simulink model "LA_KF"  (R2022a)
settings: Solver=FixedStepAuto  StartTime=0.0  StopTime=10.0  RelTol=1e-3
values from neighbouring files (symbols this model uses):
  Arm_resistance = 2.2    [Ram_rollerm.m]
  C_scr = 1.2e3    (= 1200)    [Ram_rollerm.m]
  D = 8e-5    (= 8e-05)    [Ram_rollerm.m]
  h = l/(2*pi)    (= 0.000381971863421)    [Ram_rollerm.m]
  he = 0.05    [Ram_rollerm.m]
  J = 5.3e-5    (= 5.3e-05)    [Ram_rollerm.m]
  k = 500e6    (= 500000000)    [Ram_rollerm.m]
  Ke = 0.121    [Ram_rollerm.m]
  Km = 1e7    (= 10000000)    [Ram_rollerm.m]
  Ks = 1.8e5    (= 180000)    [Ram_rollerm.m]
  Kt = 0.121    [Ram_rollerm.m]
  La = 6.4e-3    (= 0.0064)    [Ram_rollerm.m]
  lqr_Lr = lqr(Plant.A,Plant.B,lqr_Q,lqr_R)    [Ram_rollerm.m]
  M_load = 20    [Ram_rollerm.m]
  M_scr = 2    [Ram_rollerm.m]
  mu = 0.3    [Ram_rollerm.m]
  n = 0.25    [Ram_rollerm.m]
  omega = 2*pi*rpm    (= 6.28318530718)    [Ram_rollerm.m]
  R = 0.1778    [Ram_rollerm.m]
  sysKF = ss(Plant.A-Kf*Plant.C,[Plant.B Kf],eye(7),0*[Plant.B Kf])    [Ram_rollerm.m]
  w = (wo + wf)/2    (= 0.1535)    [Ram_rollerm.m]
undefined symbols (not defined in the file or in its folder): Plant
settings Model: Creator=linda  LastModifiedBy=royka
settings DebuggingCC: UnconnectedInputMsg=warning  UnconnectedOutputMsg=warning  UnconnectedLineMsg=warning
settings RTWCC: DLArmComputeVersion=19.05

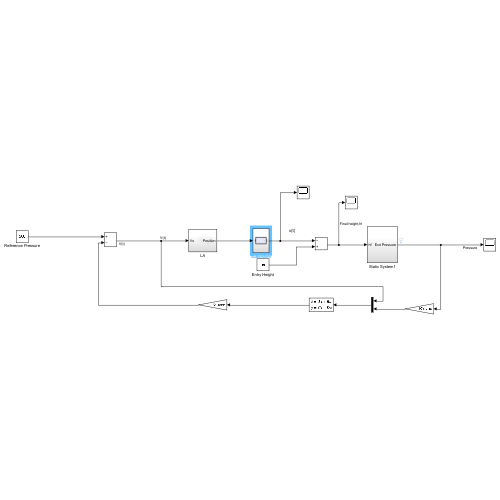
[thumbnail: Simulink's stored preview of the top-level diagram]
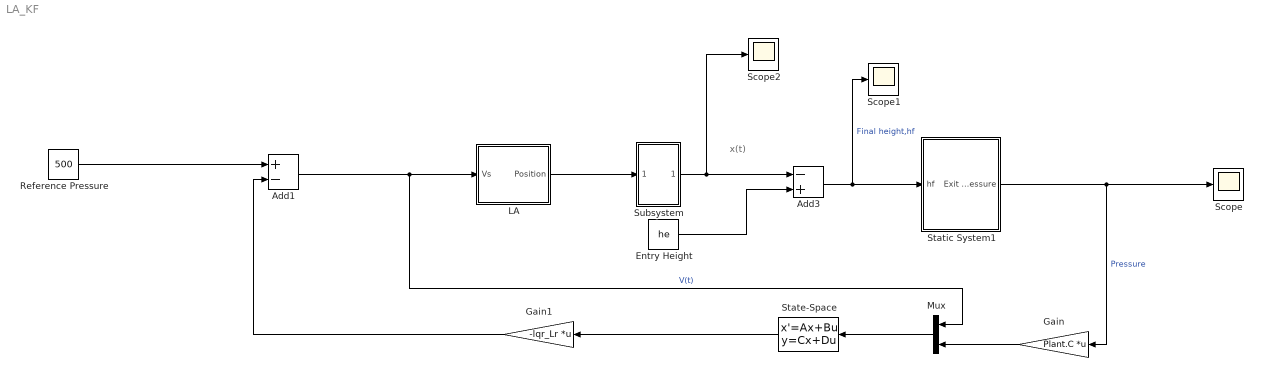
== system LA_KF ==
  note: x(t)
  Add1 : Sum  Inputs=+-
  Add3 : Sum  Inputs=-+
  Entry Height : Constant  Value=he
  Gain : Gain  Gain=Plant.C  Multiplication=Matrix(K*u) (u vector)
  Gain1 : Gain  Gain=-lqr_Lr  Multiplication=Matrix(K*u) (u vector)
  LA : Subsystem
  Mux : Mux  Inputs=2
  Reference Pressure : Constant  Value=500
  Scope : Scope
  Scope1 : Scope
  Scope2 : Scope
  State-Space : StateSpace  A=sysKF.A  B=sysKF.B  C=sysKF.C  D=sysKF.D  InitialCondition=0
  Static System1 : Subsystem
  Subsystem : Subsystem
  wires:
  Entry Height/1 -> Add3/2
  Static System1/1(Exit Pressure) -> Gain/1, Scope/1  "Pressure"
  Reference Pressure/1 -> Add1/1
  Add3/1 -> Scope1/1, Static System1/1(hf)  "Final height,hf"
  LA/1(Position) -> Subsystem/1(In1)
  Mux/1 -> State-Space/1
  Gain/1 -> Mux/2
  State-Space/1 -> Gain1/1
  Add1/1 -> LA/1(Vs), Mux/1  "V(t)"
  Gain1/1 -> Add1/2
  Subsystem/1(Out1) -> Scope2/1, Add3/1

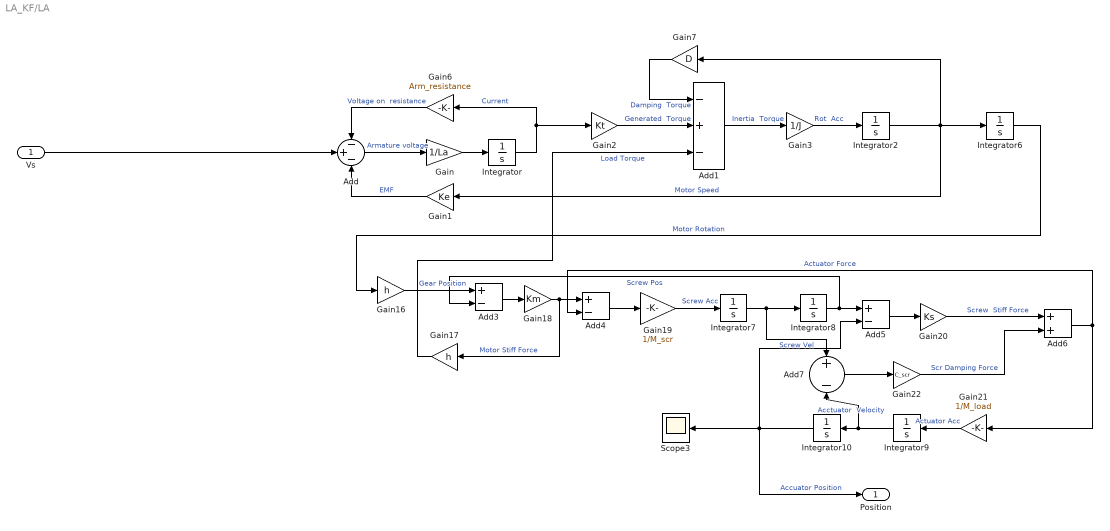
== system LA_KF/LA ==
  Vs : Inport
  Add : Sum  Inputs=-+-
  Add1 : Sum  Inputs=-+-
  Add{3..5,7} (4 alike) : Sum  Inputs=+-
  Add6 : Sum
  Gain : Gain  Gain=1/La
  Gain1 : Gain  Gain=Ke
  Gain16 : Gain  Gain=h
  Gain17 : Gain  Gain=h
  Gain18 : Gain  Gain=Km
  Gain19 : Gain  Gain=1/M_scr
  Gain2 : Gain  Gain=Kt
  Gain20 : Gain  Gain=Ks
  Gain21 : Gain  Gain=1/M_load
  Gain22 : Gain  Gain=C_scr
  Gain3 : Gain  Gain=1/J
  Gain6 : Gain  Gain=Arm_resistance
  Gain7 : Gain  Gain=D
  Integrator{,2,6..10} (7 alike) : Integrator
  Scope3 : Scope
  Position : Outport
  wires:
  Gain16/1 -> Add3/1  "Gear Position"
  Gain/1 -> Integrator/1
  Integrator8/1 -> Add3/2, Add5/1  "Screw Pos"
  Gain19/1 -> Integrator7/1  "Screw Acc"
  Gain2/1 -> Add1/2  "Generated  Torque"
  Gain20/1 -> Add6/1  "Screw  Stiff Force"
  Add1/1 -> Gain3/1  "Inertia  Torque"
  Vs/1 -> Add/2
  Gain17/1 -> Add1/3  "Load Torque"
  Gain1/1 -> Add/3  "EMF"
  Gain21/1 -> Integrator9/1  "Actuator Acc"
  Add/1 -> Gain/1  "Armature voltage"
  Add3/1 -> Gain18/1
  Gain22/1 -> Add6/2  "Scr Damping Force"
  Integrator9/1 -> Add7/2, Integrator10/1  "Acctuator  Velocity"
  Add7/1 -> Gain22/1
  Add5/1 -> Gain20/1
  Integrator/1 -> Gain6/1, Gain2/1  "Current"
  Gain6/1 -> Add/1  "Voltage on  resistance"
  Gain3/1 -> Integrator2/1  "Rot  Acc"
  Add6/1 -> Gain21/1, Add4/2  "Actuator Force"
  Integrator10/1 -> Position/1, Add5/2, Scope3/1  "Accuator Position"
  Add4/1 -> Gain19/1
  Integrator2/1 -> Gain1/1, Integrator6/1, Gain7/1  "Motor Speed"
  Integrator6/1 -> Gain16/1  "Motor Rotation"
  Gain7/1 -> Add1/1  "Damping  Torque"
  Integrator7/1 -> Add7/1, Integrator8/1  "Screw Vel"
  Gain18/1 -> Gain17/1, Add4/1  "Motor Stiff Force"

== system LA_KF/Static System1 ==
  hf : Inport
  Constant10 : Constant  Value=omega
  Subsystem : Subsystem
  Exit Pressure : Outport
  wires:
  hf/1 -> Subsystem/2(hf)  "hf"
  Constant10/1 -> Subsystem/1(omega)
  Subsystem/1(Out1) -> Exit Pressure/1

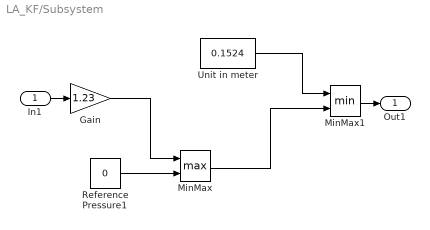
== system LA_KF/Subsystem ==
  In1 : Inport
  "Gain " : Gain  Gain=1.23
  MinMax : MinMax  Function=max  Inputs=2
  MinMax1 : MinMax  Inputs=2
  Reference Pressure1 : Constant  Value=0
  Unit in meter : Constant  Value=0.1524
  Out1 : Outport
  wires:
  MinMax1/1 -> Out1/1
  "Gain "/1 -> MinMax/1
  MinMax/1 -> MinMax1/2
  Unit in meter/1 -> MinMax1/1
  Reference Pressure1/1 -> MinMax/2
  In1/1 -> "Gain "/1

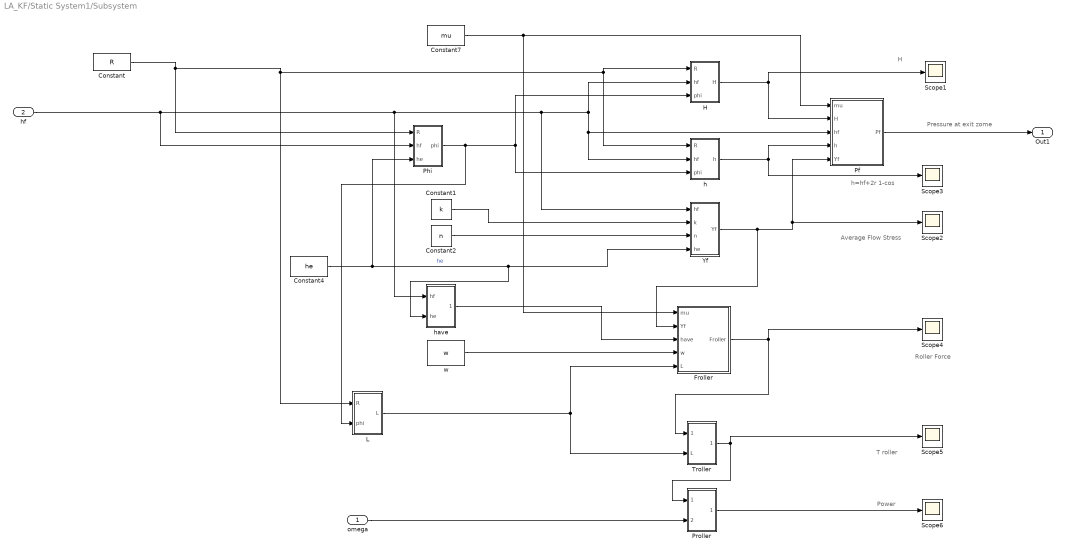
== system LA_KF/Static System1/Subsystem ==
  note: Power
  note: T roller
  note: Roller Force
  note: Pressure at exit zome
  note: h=hf+2r 1-cos
  note: Average Flow Stress
  note: H
  omega : Inport
  hf : Inport  Port=2
  Constant : Constant  Value=R
  Constant1 : Constant  Value=k
  Constant2 : Constant  Value=n
  Constant4 : Constant  Value=he
  Constant7 : Constant  Value=mu
  Froller : Subsystem
  H : Subsystem
  L : Subsystem
  Pf : Subsystem
  Phi : Subsystem
  Proller : Subsystem
  Scope{1..6} (6 alike) : Scope
  Troller : Subsystem
  Yf : Subsystem
  h : Subsystem
  have : Subsystem
  w : Constant  Value=w
  Out1 : Outport
  wires:
  omega/1 -> Proller/2(In2)
  hf/1 -> Phi/2(hf), Yf/1(hf), h/2(hf), Pf/3(hf), H/2(hf), have/1(hf)
  Yf/1(Yf) -> Froller/2(Yf), Scope2/1, Pf/5(Yf)
  Constant7/1 -> Froller/1(mu), Pf/1(mu)
  Proller/1(Out1) -> Scope6/1
  Constant4/1 -> Phi/3(he), have/2(he), Yf/4(he)  "he"
  h/1(h) -> Scope3/1, Pf/4(h)
  H/1(H) -> Scope1/1, Pf/2(H)
  w/1 -> Froller/4(w)
  Troller/1(Troller) -> Proller/1(In1), Scope5/1
  Constant2/1 -> Yf/3(n)
  Constant1/1 -> Yf/2(k)
  Froller/1(Froller) -> Scope4/1, Troller/1(Froller)
  Constant/1 -> Phi/1(R), L/1(R), H/1(R), h/1(R)
  Pf/1(Pf) -> Out1/1
  have/1(Out1) -> Froller/3(have)
  Phi/1(phi) -> L/2(phi), h/3(phi), H/3(phi)
  L/1(L) -> Troller/2(L), Froller/5(L)

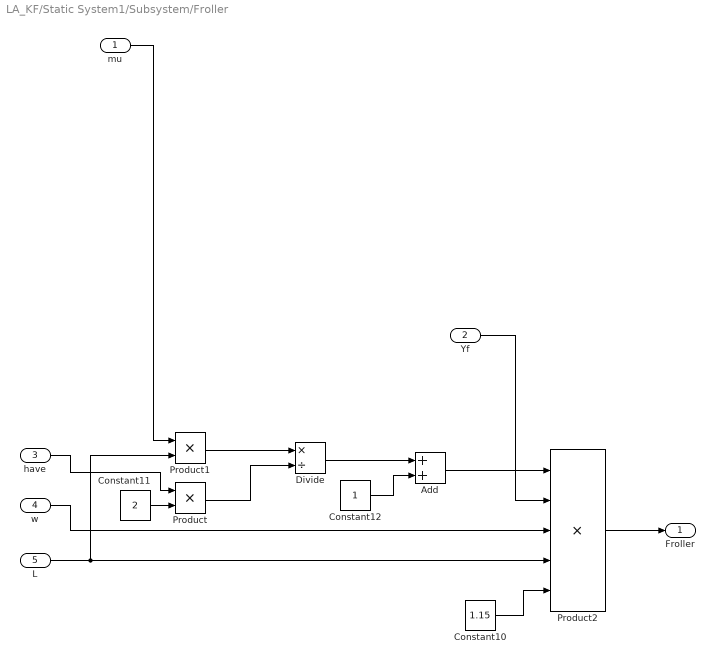
== system LA_KF/Static System1/Subsystem/Froller ==
  mu : Inport
  Yf : Inport  Port=2
  have : Inport  Port=3
  w : Inport  Port=4
  L : Inport  Port=5
  Add : Sum
  Constant10 : Constant  Value=1.15
  Constant11 : Constant  Value=2
  Constant12 : Constant
  Divide : Product  Inputs=*/
  Product : Product
  Product1 : Product
  Product2 : Product  Inputs=5
  Froller : Outport
  wires:
  L/1 -> Product2/4, Product1/2
  Product1/1 -> Divide/1
  Divide/1 -> Add/1
  Constant10/1 -> Product2/5
  Product2/1 -> Froller/1
  Constant12/1 -> Add/2
  Product/1 -> Divide/2
  Add/1 -> Product2/1
  w/1 -> Product2/3
  Constant11/1 -> Product/2
  mu/1 -> Product1/1
  Yf/1 -> Product2/2
  have/1 -> Product/1

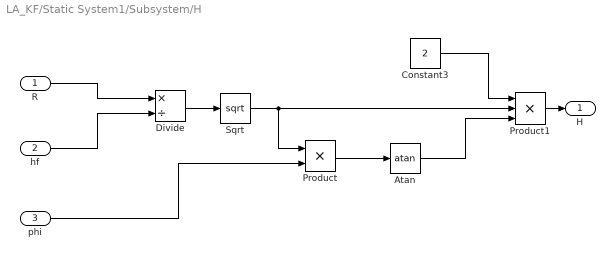
== system LA_KF/Static System1/Subsystem/H ==
  R : Inport
  hf : Inport  Port=2
  phi : Inport  Port=3
  Atan : Trigonometry  Operator=atan
  Constant3 : Constant  Value=2
  Divide : Product  Inputs=*/
  Product : Product
  Product1 : Product  Inputs=3
  Sqrt : Sqrt
  H : Outport
  wires:
  Atan/1 -> Product1/3
  Sqrt/1 -> Product/1, Product1/2
  hf/1 -> Divide/2
  Product1/1 -> H/1
  phi/1 -> Product/2
  Divide/1 -> Sqrt/1
  Product/1 -> Atan/1
  R/1 -> Divide/1
  Constant3/1 -> Product1/1

== system LA_KF/Static System1/Subsystem/L ==
  R : Inport
  phi : Inport  Port=2
  Product : Product
  L : Outport
  wires:
  Product/1 -> L/1
  phi/1 -> Product/2
  R/1 -> Product/1

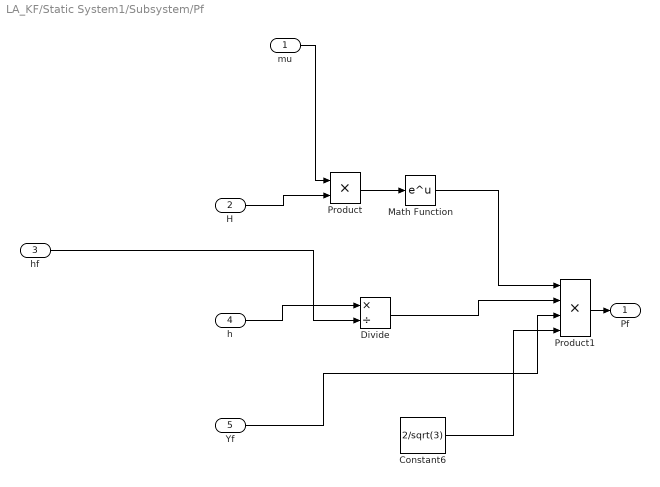
== system LA_KF/Static System1/Subsystem/Pf ==
  mu : Inport
  H : Inport  Port=2
  hf : Inport  Port=3
  h : Inport  Port=4
  Yf : Inport  Port=5
  Constant6 : Constant  Value=2/sqrt(3)
  Divide : Product  Inputs=*/
  Math Function : Math
  Product : Product
  Product1 : Product  Inputs=4
  Pf : Outport
  wires:
  h/1 -> Divide/1
  Divide/1 -> Product1/2
  Constant6/1 -> Product1/4
  Product/1 -> Math Function/1
  Yf/1 -> Product1/3
  Math Function/1 -> Product1/1
  Product1/1 -> Pf/1
  hf/1 -> Divide/2
  mu/1 -> Product/1
  H/1 -> Product/2

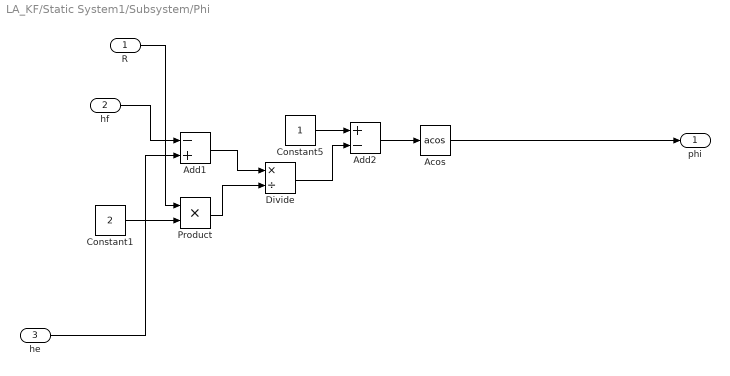
== system LA_KF/Static System1/Subsystem/Phi ==
  R : Inport
  hf : Inport  Port=2
  he : Inport  Port=3
  Acos : Trigonometry  Operator=acos
  Add1 : Sum  Inputs=-+
  Add2 : Sum  Inputs=+-
  Constant1 : Constant  Value=2
  Constant5 : Constant
  Divide : Product  Inputs=*/
  Product : Product
  phi : Outport
  wires:
  he/1 -> Add1/2
  Add1/1 -> Divide/1
  Constant1/1 -> Product/2
  Product/1 -> Divide/2
  Divide/1 -> Add2/2
  Constant5/1 -> Add2/1
  hf/1 -> Add1/1
  Add2/1 -> Acos/1
  Acos/1 -> phi/1
  R/1 -> Product/1

== system LA_KF/Static System1/Subsystem/Proller ==
  In1 : Inport
  In2 : Inport  Port=2
  Product : Product
  Out1 : Outport
  wires:
  Product/1 -> Out1/1
  In2/1 -> Product/2
  In1/1 -> Product/1

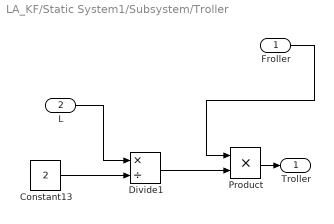
== system LA_KF/Static System1/Subsystem/Troller ==
  Froller : Inport
  L : Inport  Port=2
  Constant13 : Constant  Value=2
  Divide1 : Product  Inputs=*/
  Product : Product
  Troller : Outport
  wires:
  Divide1/1 -> Product/2
  Constant13/1 -> Divide1/2
  Froller/1 -> Product/1
  Product/1 -> Troller/1
  L/1 -> Divide1/1

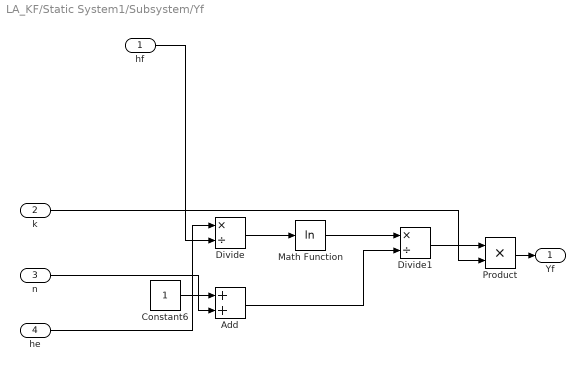
== system LA_KF/Static System1/Subsystem/Yf ==
  hf : Inport
  k : Inport  Port=2
  n : Inport  Port=3
  he : Inport  Port=4
  Add : Sum
  Constant6 : Constant
  Divide : Product  Inputs=*/
  Divide1 : Product  Inputs=*/
  Math Function : Math  Operator=log
  Product : Product
  Yf : Outport
  wires:
  n/1 -> Add/2
  Math Function/1 -> Divide1/1
  Product/1 -> Yf/1
  Divide/1 -> Math Function/1
  he/1 -> Divide/1
  Add/1 -> Divide1/2
  k/1 -> Product/2
  Constant6/1 -> Add/1
  Divide1/1 -> Product/1
  hf/1 -> Divide/2

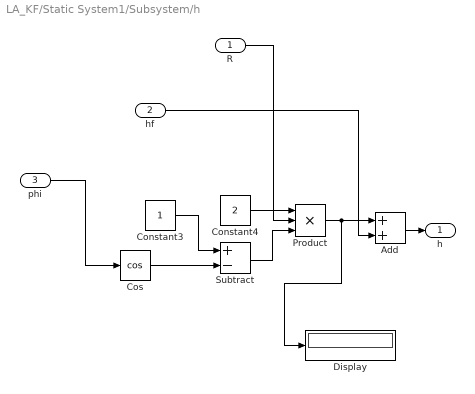
== system LA_KF/Static System1/Subsystem/h ==
  R : Inport
  hf : Inport  Port=2
  phi : Inport  Port=3
  Add : Sum
  Constant3 : Constant
  Constant4 : Constant  Value=2
  Cos : Trigonometry  Operator=cos
  Display : Display
  Product : Product  Inputs=3
  Subtract : Sum  Inputs=+-
  h : Outport
  wires:
  Add/1 -> h/1
  Subtract/1 -> Product/3
  Constant4/1 -> Product/1
  Constant3/1 -> Subtract/1
  Cos/1 -> Subtract/2
  Product/1 -> Display/1, Add/1
  phi/1 -> Cos/1
  hf/1 -> Add/2
  R/1 -> Product/2

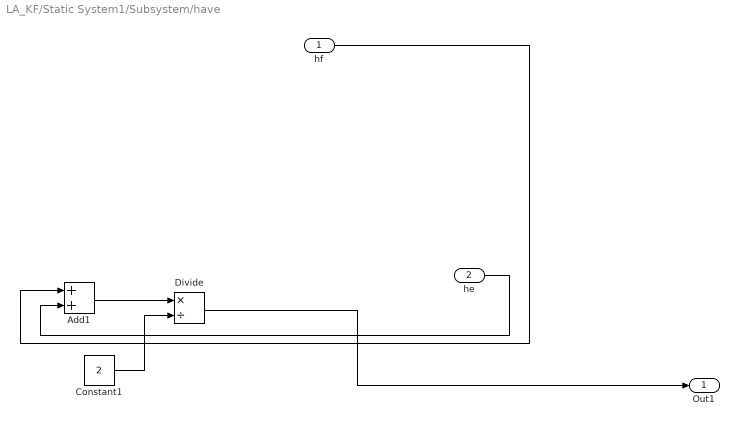
== system LA_KF/Static System1/Subsystem/have ==
  hf : Inport
  he : Inport  Port=2
  Add1 : Sum
  Constant1 : Constant  Value=2
  Divide : Product  Inputs=*/
  Out1 : Outport
  wires:
  Constant1/1 -> Divide/2
  Add1/1 -> Divide/1
  Divide/1 -> Out1/1
  he/1 -> Add1/2
  hf/1 -> Add1/1
